simulink model "Inverse_Stewart_Platform_CMM"  (R2024b)
settings: Solver=VariableStepAuto  StartTime=0.0  StopTime=0  RelTol=1e-3
settings Model: Creator=Challa  LastModifiedBy=kodan

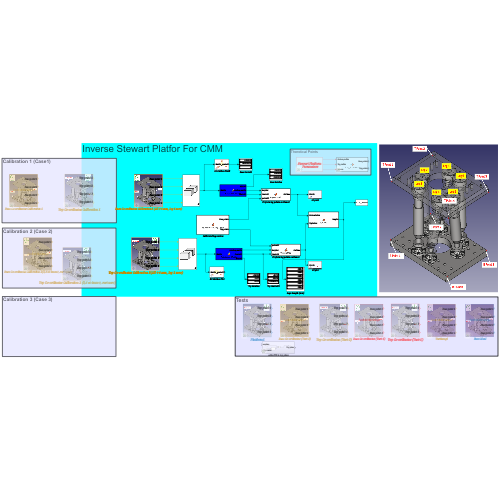
[thumbnail: Simulink's stored preview of the top-level diagram]
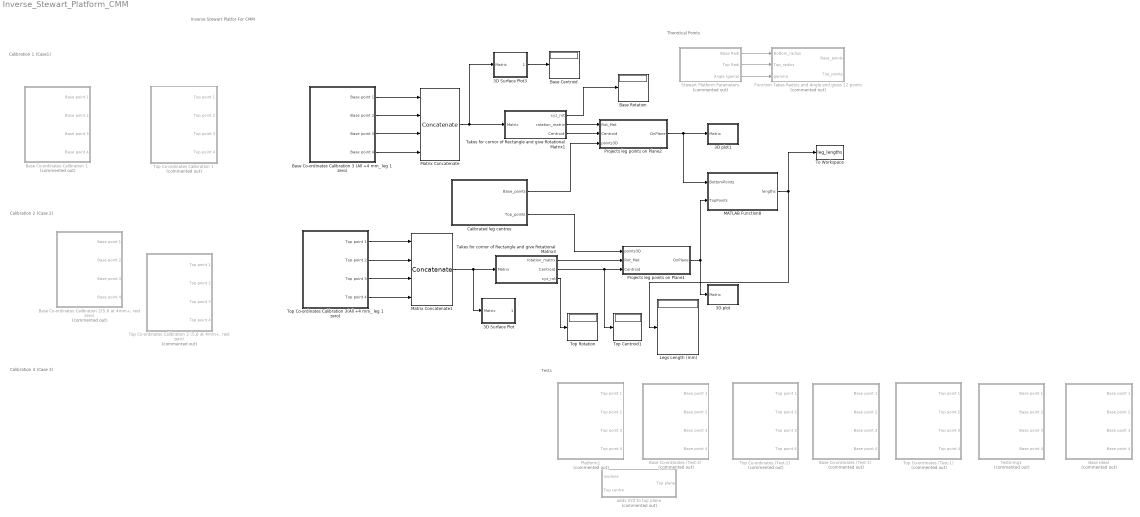
== system Inverse_Stewart_Platform_CMM ==
  note: Therotical Points
  note: Calibration 3 (Case 3)
  note: Inverse Stewart Platfor For CMM
  note: Tests
  note: Calibration 1 (Case1)
  note: Calibration 2 (Case 2)
  3D Surface Plot : Subsystem  mask(3D Surface Plot){color2='r'}
      mask prompts: color2 "color"
      mask help:
      | Input: 3xN matrix
      | output: 3D Surface Plot
      | Color: Changable by giving input
      | Finds Centerpoint and plots.
      mask Help:
      | Input: 3xN matrix
      | output: 3D Surface Plot
      | Color: Changable by giving input
      | Finds Centerpoint and plots.
      mask Display: image('XYZ2.png');
  3D Surface Plot3 : Subsystem  mask(3D Surface Plot){color2='b'}
      mask prompts: color2 "color"
      mask help:
      | Input: 3xN matrix
      | output: 3D Surface Plot
      | Color: Changable by giving input
      | Finds Centerpoint and plots.
      mask Help:
      | Input: 3xN matrix
      | output: 3D Surface Plot
      | Color: Changable by giving input
      | Finds Centerpoint and plots.
      mask Display: image('XYZ2.png');
  3D plot : Subsystem  mask(3D Plot){color1='r'}
      mask prompts: color1 "color"
      mask help:
      | Input: 3xN matrix
      | output: 3D Plot
      | Color: Changable by giving input
      mask Help:
      | Input: 3xN matrix
      | output: 3D Plot
      | Color: Changable by giving input
      mask Display: image('XYZ.png');
  3D plot1 : Subsystem  mask(3D Plot){color1='b'}
      mask prompts: color1 "color"
      mask help:
      | Input: 3xN matrix
      | output: 3D Plot
      | Color: Changable by giving input
      mask Help:
      | Input: 3xN matrix
      | output: 3D Plot
      | Color: Changable by giving input
      mask Display: image('XYZ.png');
  Base Centroid : Display
  Base Co-ordinates (Test-1) : Subsystem  Commented=on  mask(Bottom / Base platform points){B1=[-82.482,112.493,-0.004], B2=[ 82.46,112.505,0.137], B3=[82.505,-112.49,0.004], B4=[-82.482,-112.507,-0.137]}
      mask prompts: B1 "Point 1 [X Y Z] (mm)"; B2 "Point 2 [X Y Z] (mm)"; B3 "Point 3 [X Y Z] (mm)"; B4 "Point 4 [X Y Z] (mm)"
      mask help:
      | Please look at diagram to give Bottom / Base platform points
      | Array [X Y Z] with respect to the Base platform Rectangle centre
      mask Help:
      | Please look at diagram to give Bottom / Base platform points
      | Array [X Y Z] with respect to the Base platform Rectangle centre
      mask Display:
      | disp('Look at the image');
      | image('Screenshot 2024-06-21 170647.png');
  Base Co-ordinates (Test-2) : Subsystem  Commented=on  mask(Bottom / Base platform points){B1=[-82.482,112.494,0.006], B2=[82.459,112.506,0.136], B3=[82.506,-112.491,-0.006], B4=[-82.482,-112.508,-0.136]}
      mask prompts: B1 "Point 1 [X Y Z] (mm)"; B2 "Point 2 [X Y Z] (mm)"; B3 "Point 3 [X Y Z] (mm)"; B4 "Point 4 [X Y Z] (mm)"
      mask help:
      | Please look at diagram to give Bottom / Base platform points
      | Array [X Y Z] with respect to the Base platform Rectangle centre
      mask Help:
      | Please look at diagram to give Bottom / Base platform points
      | Array [X Y Z] with respect to the Base platform Rectangle centre
      mask Display:
      | disp('Look at the image');
      | image('Screenshot 2024-06-21 170647.png');
  Base Co-ordinates Calibration 1 : Subsystem  Commented=on  mask(Bottom / Base platform points){B1=[-82.478,112.495,-0.004], B2=[82.454,112.508,0.112], B3=[82.502,-112.489,0.004], B4=[-82.478,-112.513,-0.112]}
      mask prompts: B1 "Point 1 [X Y Z] (mm)"; B2 "Point 2 [X Y Z] (mm)"; B3 "Point 3 [X Y Z] (mm)"; B4 "Point 4 [X Y Z] (mm)"
      mask help:
      | Please look at diagram to give Bottom / Base platform points
      | Array [X Y Z] with respect to the Base platform Rectangle centre
      mask Help:
      | Please look at diagram to give Bottom / Base platform points
      | Array [X Y Z] with respect to the Base platform Rectangle centre
      mask Display:
      | disp('Look at the image');
      | image('Screenshot 2024-06-21 170647.png');
  "Base Co-ordinates Calibration 2(5,6 at 4mm+, rest zero)" : Subsystem  Commented=on  mask(Bottom / Base platform points){B1=[-82.477,112.496,-0.004], B2=[82.452,112.506,0.125], B3=[82.503,-112.49,0.004], B4=[-82.477,-112.511,-0.125]}
      mask prompts: B1 "Point 1 [X Y Z] (mm)"; B2 "Point 2 [X Y Z] (mm)"; B3 "Point 3 [X Y Z] (mm)"; B4 "Point 4 [X Y Z] (mm)"
      mask help:
      | Please look at diagram to give Bottom / Base platform points
      | Array [X Y Z] with respect to the Base platform Rectangle centre
      mask Help:
      | Please look at diagram to give Bottom / Base platform points
      | Array [X Y Z] with respect to the Base platform Rectangle centre
      mask Display:
      | disp('Look at the image');
      | image('Screenshot 2024-06-21 170647.png');
  Base Co-ordinates Calibration 3 (All +4 mm_ leg 1 zero) : Subsystem  mask(Bottom / Base platform points){B1=[-82.477,112.497,-0.008], B2=[82.453,112.508,0.126], B3=[82.502,-112.492,0.008], B4=[-82.477,-112.513,-0.126]}
      mask prompts: B1 "Point 1 [X Y Z] (mm)"; B2 "Point 2 [X Y Z] (mm)"; B3 "Point 3 [X Y Z] (mm)"; B4 "Point 4 [X Y Z] (mm)"
      mask help:
      | Please look at diagram to give Bottom / Base platform points
      | Array [X Y Z] with respect to the Base platform Rectangle centre
      mask Help:
      | Please look at diagram to give Bottom / Base platform points
      | Array [X Y Z] with respect to the Base platform Rectangle centre
      mask Display:
      | disp('Look at the image');
      | image('Screenshot 2024-06-21 170647.png');
  Base Ideal : Subsystem  Commented=on  mask(Bottom / Base platform points){B1=[-82.5,112.5,0], B2=[82.5,112.5,0], B3=[82.5,-112.5,0], B4=[-82.5,-112.5,0]}
      mask prompts: B1 "Point 1 [X Y Z] (mm)"; B2 "Point 2 [X Y Z] (mm)"; B3 "Point 3 [X Y Z] (mm)"; B4 "Point 4 [X Y Z] (mm)"
      mask help:
      | Please look at diagram to give Bottom / Base platform points
      | Array [X Y Z] with respect to the Base platform Rectangle centre
      mask Help:
      | Please look at diagram to give Bottom / Base platform points
      | Array [X Y Z] with respect to the Base platform Rectangle centre
      mask Display:
      | disp('Look at the image');
      | image('Screenshot 2024-06-21 170647.png');
  Base Rotation : Display
  Calibrated leg centres : MATLAB Function  TreatAsAtomicUnit=on
  Function Takes Radius and Angle and gives 12 points : MATLAB Function  Commented=on  TreatAsAtomicUnit=on
  Legs Length (mm) : Display
  MATLAB Function8 : MATLAB Function  TreatAsAtomicUnit=on
  Matrix Concatenate : Concatenate  NumInputs=4  Mode=Multidimensional array  ConcatenateDimension=2
  Matrix Concatenate1 : Concatenate  NumInputs=4  Mode=Multidimensional array  ConcatenateDimension=2
  Platform1 : Subsystem  Commented=on  mask(Top / Moving Platform Points){T1=|, T2=|, T3=|, T4=|}
      mask T1=|
      | [-122.0492
      | 96.5349
      | 168.8901]
      mask T2=|
      | [27.7169
      | 145.1424
      | 218.2097]
      mask T3=|
      | [102.0492
      | -66.5349
      | 201.1099]
      mask T4=|
      | [-47.7169
      | -115.1424
      | 151.7903]
      mask prompts: T1 "Point 1 [X Y Z] (mm)"; T2 "Point 2 [X Y Z] (mm)"; T3 "Point 3 [X Y Z] (mm)"; T4 "Point 4 [X Y Z] (mm)"
      mask help:
      | Please look at diagram to give Top / Moving Platform points
      | Array [X Y Z] with respect to the Base platform Rectangle centre
      mask Help:
      | Please look at diagram to give Top / Moving Platform points
      | Array [X Y Z] with respect to the Base platform Rectangle centre
      mask Display: image('Screenshot 2024-06-21 172342.png');
  Projects leg points on Plane1 : MATLAB Function  TreatAsAtomicUnit=on
  Projects leg points on Plane2 : MATLAB Function  TreatAsAtomicUnit=on
  Stewart Platform Parameters : Subsystem  Commented=on  mask(Gamma or Angle){B_R=130/2, T_R=125/2, Angle=20}
      mask prompts: B_R "Base Radius (mm)"; T_R "Top Radius(mm)"; Angle "Angle or Gama(deg)"
      mask help: Gamma is the half angle between 2 centres of leg
      mask Help: Gamma is the half angle between 2 centres of leg
      mask Display: disp('Stewart Platform \n Paramaters');
  Takes for cornor of Rectangle and give Rotational Matrix1 : MATLAB Function  TreatAsAtomicUnit=on
  Takes for cornor of Rectangle and give Rotational Matrix3 : MATLAB Function  TreatAsAtomicUnit=on
  Testinmg1 : Subsystem  Commented=on  mask(Bottom / Base platform points){B1=[-82.5,112.5,185], B2=[82.5,112.5,185], B3=[82.5,-112.5,185], B4=[-82.5,-112.5,185]}
      mask prompts: B1 "Point 1 [X Y Z] (mm)"; B2 "Point 2 [X Y Z] (mm)"; B3 "Point 3 [X Y Z] (mm)"; B4 "Point 4 [X Y Z] (mm)"
      mask help:
      | Please look at diagram to give Bottom / Base platform points
      | Array [X Y Z] with respect to the Base platform Rectangle centre
      mask Help:
      | Please look at diagram to give Bottom / Base platform points
      | Array [X Y Z] with respect to the Base platform Rectangle centre
      mask Display:
      | disp('Look at the image');
      | image('Screenshot 2024-06-21 170647.png');
  To Workspace : ToWorkspace  VariableName=leg_lengths  SampleTime=-1
      settings: Save2DSignal=2-D array (concatenate along first dimension)
  Top Centroid1 : Display
  Top Co-ordinates (Test-1) : Subsystem  Commented=on  mask(Top / Moving Platform Points){T1=[-83.589,104.282,181.898], T2=[ 81.27,109.355,180.899], T3=[88.271,-115.398,175.913], T4=[-76.576,-120.558,176.91]}
      mask prompts: T1 "Point 1 [X Y Z] (mm)"; T2 "Point 2 [X Y Z] (mm)"; T3 "Point 3 [X Y Z] (mm)"; T4 "Point 4 [X Y Z] (mm)"
      mask help:
      | Please look at diagram to give Top / Moving Platform points
      | Array [X Y Z] with respect to the Base platform Rectangle centre
      mask Help:
      | Please look at diagram to give Top / Moving Platform points
      | Array [X Y Z] with respect to the Base platform Rectangle centre
      mask Display: image('Screenshot 2024-06-21 172342.png');
  Top Co-ordinates (Test-2) : Subsystem  Commented=on  mask(Top / Moving Platform Points){T1=[-88.819,113.319,179.407], T2=[ 76.042,118.442,180.272], T3=[83.131,-106.372,180.49], T4=[-81.723,-111.564,179.625]}
      mask prompts: T1 "Point 1 [X Y Z] (mm)"; T2 "Point 2 [X Y Z] (mm)"; T3 "Point 3 [X Y Z] (mm)"; T4 "Point 4 [X Y Z] (mm)"
      mask help:
      | Please look at diagram to give Top / Moving Platform points
      | Array [X Y Z] with respect to the Base platform Rectangle centre
      mask Help:
      | Please look at diagram to give Top / Moving Platform points
      | Array [X Y Z] with respect to the Base platform Rectangle centre
      mask Display: image('Screenshot 2024-06-21 172342.png');
  Top Co-ordinates Calibration 1 : Subsystem  Commented=on  mask(Top / Moving Platform Points){T1=[-78.089,115.325,180.165], T2=[86.773,110.209,179.929], T3=[79.912,-114.609,179.521], T4=[-84.943,-109.583,179.756]}
      mask prompts: T1 "Point 1 [X Y Z] (mm)"; T2 "Point 2 [X Y Z] (mm)"; T3 "Point 3 [X Y Z] (mm)"; T4 "Point 4 [X Y Z] (mm)"
      mask help:
      | Please look at diagram to give Top / Moving Platform points
      | Array [X Y Z] with respect to the Base platform Rectangle centre
      mask Help:
      | Please look at diagram to give Top / Moving Platform points
      | Array [X Y Z] with respect to the Base platform Rectangle centre
      mask Display: image('Screenshot 2024-06-21 172342.png');
  "Top Co-ordinates Calibration 2 (5,6 at 4mm+, rest zero)" : Subsystem  Commented=on  mask(Top / Moving Platform Points){T1=[-85.125,127.502,176.101], T2=[79.718,122.365,179.083], T3=[72.703,-102.365,185.192], T4=[-92.131,-97.306,182.212]}
      mask prompts: T1 "Point 1 [X Y Z] (mm)"; T2 "Point 2 [X Y Z] (mm)"; T3 "Point 3 [X Y Z] (mm)"; T4 "Point 4 [X Y Z] (mm)"
      mask help:
      | Please look at diagram to give Top / Moving Platform points
      | Array [X Y Z] with respect to the Base platform Rectangle centre
      mask Help:
      | Please look at diagram to give Top / Moving Platform points
      | Array [X Y Z] with respect to the Base platform Rectangle centre
      mask Display: image('Screenshot 2024-06-21 172342.png');
  Top Co-ordinates Calibration 3(All +4 mm_ leg 1 zero) : Subsystem  mask(Top / Moving Platform Points){T1=[-91.542,118.596,184.014], T2=[73.104,127.707,179.994], T3=[85.709,-96.849,181.665], T4=[-78.923,-106.062,185.686]}
      mask prompts: T1 "Point 1 [X Y Z] (mm)"; T2 "Point 2 [X Y Z] (mm)"; T3 "Point 3 [X Y Z] (mm)"; T4 "Point 4 [X Y Z] (mm)"
      mask help:
      | Please look at diagram to give Top / Moving Platform points
      | Array [X Y Z] with respect to the Base platform Rectangle centre
      mask Help:
      | Please look at diagram to give Top / Moving Platform points
      | Array [X Y Z] with respect to the Base platform Rectangle centre
      mask Display: image('Screenshot 2024-06-21 172342.png');
  Top Rotation : Display
  adds XYZ to top plane : Subsystem  Commented=on
  wires:
  Matrix Concatenate1/1 -> 3D Surface Plot/1(Matrix), Takes for cornor of Rectangle and give Rotational Matrix3/1(Matrix)
  Top Co-ordinates Calibration 3(All +4 mm_ leg 1 zero)/4(Top point 4) -> Matrix Concatenate1/4
  Top Co-ordinates Calibration 3(All +4 mm_ leg 1 zero)/3(Top point 3) -> Matrix Concatenate1/3
  Takes for cornor of Rectangle and give Rotational Matrix1/2(rotation_matrix) -> Projects leg points on Plane2/1(Rot_Mat)
  Top Co-ordinates Calibration 3(All +4 mm_ leg 1 zero)/2(Top point 2) -> Matrix Concatenate1/2
  Takes for cornor of Rectangle and give Rotational Matrix1/3(Centroid) -> Projects leg points on Plane2/2(Centroid)
  Top Co-ordinates Calibration 3(All +4 mm_ leg 1 zero)/1(Top point 1) -> Matrix Concatenate1/1
  Stewart Platform Parameters/3(Angle (gama)) -> Function Takes Radius and Angle and gives 12 points/3(gamma)
  Stewart Platform Parameters/2(Top Radi) -> Function Takes Radius and Angle and gives 12 points/2(Top_radius)
  Stewart Platform Parameters/1(Base Radi) -> Function Takes Radius and Angle and gives 12 points/1(Bottom_radius)
  Calibrated leg centres/1(Base_points) -> Projects leg points on Plane2/3(points3D)
  Calibrated leg centres/2(Top_points) -> Projects leg points on Plane1/1(points3D)
  3D Surface Plot3/1(centroid) -> Base Centroid/1
  Takes for cornor of Rectangle and give Rotational Matrix3/1(rotation_matrix) -> Projects leg points on Plane1/2(Rot_Mat)
  Takes for cornor of Rectangle and give Rotational Matrix3/2(Centroid) -> Projects leg points on Plane1/3(Centroid), Top Centroid1/1
  Base Co-ordinates Calibration 3 (All +4 mm_ leg 1 zero)/4(Base point 4) -> Matrix Concatenate/4
  Takes for cornor of Rectangle and give Rotational Matrix3/3(xyz_rot) -> Top Rotation/1
  Projects leg points on Plane2/1(OnPlane) -> MATLAB Function8/1(BottomPoints), 3D plot1/1(Matrix)
  Projects leg points on Plane1/1(OnPlane) -> MATLAB Function8/2(TopPoints), 3D plot/1(Matrix)
  MATLAB Function8/1(lengths) -> Legs Length (mm)/1, To Workspace/1
  Base Co-ordinates Calibration 3 (All +4 mm_ leg 1 zero)/1(Base point 1) -> Matrix Concatenate/1
  Base Co-ordinates Calibration 3 (All +4 mm_ leg 1 zero)/2(Base point 2) -> Matrix Concatenate/2
  Base Co-ordinates Calibration 3 (All +4 mm_ leg 1 zero)/3(Base point 3) -> Matrix Concatenate/3
  Matrix Concatenate/1 -> 3D Surface Plot3/1(Matrix), Takes for cornor of Rectangle and give Rotational Matrix1/1(Matrix)
  Takes for cornor of Rectangle and give Rotational Matrix1/1(xyz_rot) -> Base Rotation/1

== system Inverse_Stewart_Platform_CMM/3D Surface Plot ==
  Matrix : Inport
  MATLAB Function6 : MATLAB Function  TreatAsAtomicUnit=on
  Plot3D1 : MATLAB Function  TreatAsAtomicUnit=on
  Plot3D6 : MATLAB Function  TreatAsAtomicUnit=on
  String Constant : StringConstant  String=color2
  centroid : Outport
  wires:
  Matrix/1 -> Plot3D1/1(Matrix), MATLAB Function6/1(Matrix)
  MATLAB Function6/1(centroid) -> centroid/1, Plot3D6/1(Matrix)
  String Constant/1 -> Plot3D6/2(color2), Plot3D1/2(color2)

== system Inverse_Stewart_Platform_CMM/3D Surface Plot3 ==
  Matrix : Inport
  MATLAB Function6 : MATLAB Function  TreatAsAtomicUnit=on
  Plot3D1 : MATLAB Function  TreatAsAtomicUnit=on
  Plot3D6 : MATLAB Function  TreatAsAtomicUnit=on
  String Constant : StringConstant  String=color2
  centroid : Outport
  wires:
  String Constant/1 -> Plot3D1/2(color2), Plot3D6/2(color2)
  MATLAB Function6/1(centroid) -> Plot3D6/1(Matrix), centroid/1
  Matrix/1 -> MATLAB Function6/1(Matrix), Plot3D1/1(Matrix)

== system Inverse_Stewart_Platform_CMM/3D plot ==
  Matrix : Inport
  Plot3D1 : MATLAB Function  TreatAsAtomicUnit=on
  String Constant : StringConstant  String=color1
  wires:
  String Constant/1 -> Plot3D1/2(color1)
  Matrix/1 -> Plot3D1/1(Matrix)

== system Inverse_Stewart_Platform_CMM/3D plot1 ==
  Matrix : Inport
  Plot3D1 : MATLAB Function  TreatAsAtomicUnit=on
  String Constant : StringConstant  String=color1
  wires:
  Matrix/1 -> Plot3D1/1(Matrix)
  String Constant/1 -> Plot3D1/2(color1)

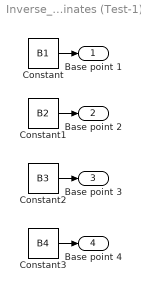
== system Inverse_Stewart_Platform_CMM/Base Co-ordinates (Test-1) ==
  Constant : Constant  Value=B1
  Constant1 : Constant  Value=B2
  Constant2 : Constant  Value=B3
  Constant3 : Constant  Value=B4
  Base point 1 : Outport
  Base point 2 : Outport  Port=2
  Base point 3 : Outport  Port=3
  Base point 4 : Outport  Port=4
  wires:
  Constant1/1 -> Base point 2/1
  Constant3/1 -> Base point 4/1
  Constant2/1 -> Base point 3/1
  Constant/1 -> Base point 1/1

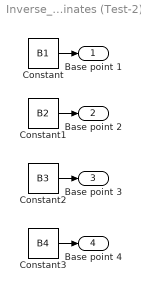
== system Inverse_Stewart_Platform_CMM/Base Co-ordinates (Test-2) ==
  Constant : Constant  Value=B1
  Constant1 : Constant  Value=B2
  Constant2 : Constant  Value=B3
  Constant3 : Constant  Value=B4
  Base point 1 : Outport
  Base point 2 : Outport  Port=2
  Base point 3 : Outport  Port=3
  Base point 4 : Outport  Port=4
  wires:
  Constant1/1 -> Base point 2/1
  Constant3/1 -> Base point 4/1
  Constant2/1 -> Base point 3/1
  Constant/1 -> Base point 1/1

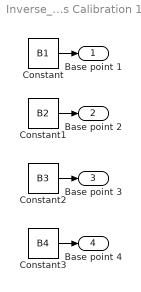
== system Inverse_Stewart_Platform_CMM/Base Co-ordinates Calibration 1 ==
  Constant : Constant  Value=B1
  Constant1 : Constant  Value=B2
  Constant2 : Constant  Value=B3
  Constant3 : Constant  Value=B4
  Base point 1 : Outport
  Base point 2 : Outport  Port=2
  Base point 3 : Outport  Port=3
  Base point 4 : Outport  Port=4
  wires:
  Constant/1 -> Base point 1/1
  Constant2/1 -> Base point 3/1
  Constant3/1 -> Base point 4/1
  Constant1/1 -> Base point 2/1

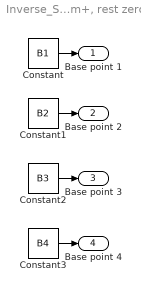
== system Inverse_Stewart_Platform_CMM/Base Co-ordinates Calibration 2(5,6 at 4mm+, rest zero) ==
  Constant : Constant  Value=B1
  Constant1 : Constant  Value=B2
  Constant2 : Constant  Value=B3
  Constant3 : Constant  Value=B4
  Base point 1 : Outport
  Base point 2 : Outport  Port=2
  Base point 3 : Outport  Port=3
  Base point 4 : Outport  Port=4
  wires:
  Constant1/1 -> Base point 2/1
  Constant3/1 -> Base point 4/1
  Constant2/1 -> Base point 3/1
  Constant/1 -> Base point 1/1

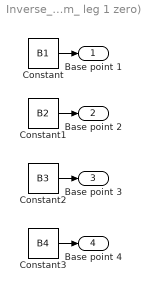
== system Inverse_Stewart_Platform_CMM/Base Co-ordinates Calibration 3 (All +4 mm_ leg 1 zero) ==
  Constant : Constant  Value=B1
  Constant1 : Constant  Value=B2
  Constant2 : Constant  Value=B3
  Constant3 : Constant  Value=B4
  Base point 1 : Outport
  Base point 2 : Outport  Port=2
  Base point 3 : Outport  Port=3
  Base point 4 : Outport  Port=4
  wires:
  Constant1/1 -> Base point 2/1
  Constant3/1 -> Base point 4/1
  Constant2/1 -> Base point 3/1
  Constant/1 -> Base point 1/1

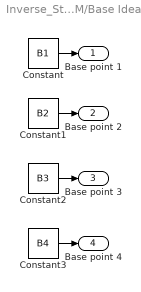
== system Inverse_Stewart_Platform_CMM/Base Ideal ==
  Constant : Constant  Value=B1
  Constant1 : Constant  Value=B2
  Constant2 : Constant  Value=B3
  Constant3 : Constant  Value=B4
  Base point 1 : Outport
  Base point 2 : Outport  Port=2
  Base point 3 : Outport  Port=3
  Base point 4 : Outport  Port=4
  wires:
  Constant/1 -> Base point 1/1
  Constant2/1 -> Base point 3/1
  Constant3/1 -> Base point 4/1
  Constant1/1 -> Base point 2/1

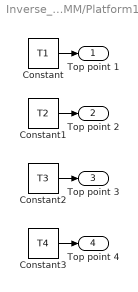
== system Inverse_Stewart_Platform_CMM/Platform1 ==
  Constant : Constant  Value=T1
  Constant1 : Constant  Value=T2
  Constant2 : Constant  Value=T3
  Constant3 : Constant  Value=T4
  Top point 1 : Outport
  Top point 2 : Outport  Port=2
  Top point 3 : Outport  Port=3
  Top point 4 : Outport  Port=4
  wires:
  Constant/1 -> Top point 1/1
  Constant2/1 -> Top point 3/1
  Constant3/1 -> Top point 4/1
  Constant1/1 -> Top point 2/1

== system Inverse_Stewart_Platform_CMM/Stewart Platform Parameters ==
  Angle : Constant  Value=Angle
  Base Radius : Constant  Value=B_R
  Top Radius : Constant  Value=T_R
  Base Radi : Outport
  Top Radi : Outport  Port=2
  Angle (gama) : Outport  Port=3
  wires:
  Angle/1 -> Angle (gama)/1
  Base Radius/1 -> Base Radi/1
  Top Radius/1 -> Top Radi/1

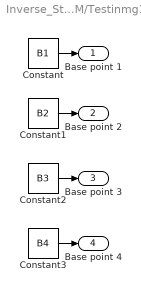
== system Inverse_Stewart_Platform_CMM/Testinmg1 ==
  Constant : Constant  Value=B1
  Constant1 : Constant  Value=B2
  Constant2 : Constant  Value=B3
  Constant3 : Constant  Value=B4
  Base point 1 : Outport
  Base point 2 : Outport  Port=2
  Base point 3 : Outport  Port=3
  Base point 4 : Outport  Port=4
  wires:
  Constant1/1 -> Base point 2/1
  Constant3/1 -> Base point 4/1
  Constant2/1 -> Base point 3/1
  Constant/1 -> Base point 1/1

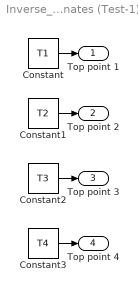
== system Inverse_Stewart_Platform_CMM/Top Co-ordinates (Test-1) ==
  Constant : Constant  Value=T1
  Constant1 : Constant  Value=T2
  Constant2 : Constant  Value=T3
  Constant3 : Constant  Value=T4
  Top point 1 : Outport
  Top point 2 : Outport  Port=2
  Top point 3 : Outport  Port=3
  Top point 4 : Outport  Port=4
  wires:
  Constant1/1 -> Top point 2/1
  Constant3/1 -> Top point 4/1
  Constant2/1 -> Top point 3/1
  Constant/1 -> Top point 1/1

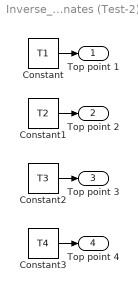
== system Inverse_Stewart_Platform_CMM/Top Co-ordinates (Test-2) ==
  Constant : Constant  Value=T1
  Constant1 : Constant  Value=T2
  Constant2 : Constant  Value=T3
  Constant3 : Constant  Value=T4
  Top point 1 : Outport
  Top point 2 : Outport  Port=2
  Top point 3 : Outport  Port=3
  Top point 4 : Outport  Port=4
  wires:
  Constant/1 -> Top point 1/1
  Constant2/1 -> Top point 3/1
  Constant3/1 -> Top point 4/1
  Constant1/1 -> Top point 2/1

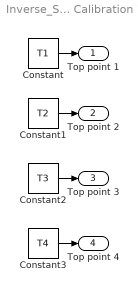
== system Inverse_Stewart_Platform_CMM/Top Co-ordinates Calibration 1 ==
  Constant : Constant  Value=T1
  Constant1 : Constant  Value=T2
  Constant2 : Constant  Value=T3
  Constant3 : Constant  Value=T4
  Top point 1 : Outport
  Top point 2 : Outport  Port=2
  Top point 3 : Outport  Port=3
  Top point 4 : Outport  Port=4
  wires:
  Constant1/1 -> Top point 2/1
  Constant3/1 -> Top point 4/1
  Constant2/1 -> Top point 3/1
  Constant/1 -> Top point 1/1

== system Inverse_Stewart_Platform_CMM/Top Co-ordinates Calibration 2 (5,6 at 4mm+, rest zero) ==
  Constant : Constant  Value=T1
  Constant1 : Constant  Value=T2
  Constant2 : Constant  Value=T3
  Constant3 : Constant  Value=T4
  Top point 1 : Outport
  Top point 2 : Outport  Port=2
  Top point 3 : Outport  Port=3
  Top point 4 : Outport  Port=4
  wires:
  Constant/1 -> Top point 1/1
  Constant2/1 -> Top point 3/1
  Constant3/1 -> Top point 4/1
  Constant1/1 -> Top point 2/1

== system Inverse_Stewart_Platform_CMM/Top Co-ordinates Calibration 3(All +4 mm_ leg 1 zero) ==
  Constant : Constant  Value=T1
  Constant1 : Constant  Value=T2
  Constant2 : Constant  Value=T3
  Constant3 : Constant  Value=T4
  Top point 1 : Outport
  Top point 2 : Outport  Port=2
  Top point 3 : Outport  Port=3
  Top point 4 : Outport  Port=4
  wires:
  Constant/1 -> Top point 1/1
  Constant2/1 -> Top point 3/1
  Constant3/1 -> Top point 4/1
  Constant1/1 -> Top point 2/1

== system Inverse_Stewart_Platform_CMM/adds XYZ to top plane ==
  onplane : Inport
  " Top centre" : Inport  Port=2
  Add : Sum
  MATLAB Function : MATLAB Function  TreatAsAtomicUnit=on
  Top plane : Outport
  wires:
  onplane/1 -> Add/1
  " Top centre"/1 -> MATLAB Function/1(u)
  Add/1 -> Top plane/1
  MATLAB Function/1(y) -> Add/2

== matlab function Inverse_Stewart_Platform_CMM/3D Surface Plot/Plot3D6 ==
  data: Matrix input; color2 input
function Plot3D(Matrix,color2)

figure(1)
x = Matrix(1, :);
y = Matrix(2, :);
z = Matrix(3, :);

% Create the 3D plot
plot3(x, y, z, 'o-', 'Color',color2,'LineWidth', 2);

xlabel('X Axis');
ylabel('Y Axis');
zlabel('Z Axis');


grid on


hold on;

% Connect the initial and final points
plot3([x(1) x(end)], [y(1) y(end)], [z(1) z(end)], 'o-', 'Color',color2,'LineWidth', 2);

%hold on

end

== matlab function Inverse_Stewart_Platform_CMM/Takes for cornor of Rectangle and give Rotational Matrix3 ==
  data: Matrix input; rotation_matrix output; Centroid output; xyz_rot output
function [rotation_matrix,Centroid, xyz_rot] = Rotational_Matrix(Matrix)
    % A, B, C, D are the 3D coordinates of the rectangle's corners

    Centroid = mean(Matrix, 2);

    A = Matrix(:,1);
    B = Matrix(:,2);
    C = Matrix(:,3);
    D = Matrix(:,4);

    % Calculate the normal vector of the plane using cross product
    AB = B - A;
    AD = A - D;
    normal = cross(AB, AD);
    normal = normal / norm(normal); % Normalize the normal vector

    % Create orthogonal basis vectors on the plane
    e1 = AB / norm(AB); % First direction vector on the plane
    e2 = cross(normal, e1); % Second direction vector on the plane

    % Construct the rotation matrix from the plane's basis vectors
    rotation_matrix = [e1 e2 normal];

    % Calculate Euler angles (rotations in XYZ)
    xyz_rot = rad2deg(rotm2eul(rotation_matrix,"XYZ"));


    % Assuming the rectangle is initially aligned with the XY plane,
    % we can calculate the rotations needed to align it with the given orientation.
    % % % % % thetaX = atan2(normal(2), normal(3));
    % % % % % thetaY = atan2(-normal(1), sqrt(normal(2)^2 + normal(3)^2));
    % % % % % thetaZ = atan2(AB(2), AB(1));
    % % % % % 
    % % % % % % Convert angles to degrees
    % % % % % thetaX_deg = rad2deg(thetaX);
    % % % % % thetaY_deg = rad2deg(thetaY);
    % % % % % thetaZ_deg = rad2deg(thetaZ);
    % % % % % xyz_rot = [thetaX_deg,thetaY_deg, thetaZ_deg];
end

== matlab function Inverse_Stewart_Platform_CMM/3D Surface Plot3/MATLAB Function6 ==
  data: Matrix input; centroid output
function centroid  = FindCentroid(Matrix)
    % This function calculates the centroid of a 3xN matrix
    % points: a 3xN matrix where each column represents a point in 3D space
    % centroid: a 3x1 vector representing the center point of the given points

    % Validate input
    if size(Matrix, 1) ~= 3
        error('Input matrix must have 3 rows');
    end

    % Calculate the centroid
    centroid = mean(Matrix, 2);
end

== matlab function Inverse_Stewart_Platform_CMM/3D Surface Plot3/Plot3D1 ==
  data: Matrix input; color2 input
function Plot3D(Matrix, color2)

figure(1)
x = Matrix(1, :);
y = Matrix(2, :);
z = Matrix(3, :);

% Create the 3D plot
plot3(x, y, z, 'o-', 'Color',color2,'LineWidth', 2);
hold on
fill3(x, y, z, color2, 'FaceAlpha', 0.2)
xlabel('X Axis');
ylabel('Y Axis');
zlabel('Z Axis');

axis equal
grid on


hold on;

% Connect the initial and final points
plot3([x(1) x(end)], [y(1) y(end)], [z(1) z(end)], 'o-', 'Color',color2,'LineWidth', 2);

hold on

end

== matlab function Inverse_Stewart_Platform_CMM/3D Surface Plot3/Plot3D6 ==
  data: Matrix input; color2 input
function Plot3D(Matrix,color2)

figure(1)
x = Matrix(1, :);
y = Matrix(2, :);
z = Matrix(3, :);

% Create the 3D plot
plot3(x, y, z, 'o-', 'Color',color2,'LineWidth', 2);
xlabel('X Axis');
ylabel('Y Axis');
zlabel('Z Axis');


grid on


hold on;

% Connect the initial and final points
plot3([x(1) x(end)], [y(1) y(end)], [z(1) z(end)], 'o-', 'Color',color2,'LineWidth', 2);

hold on

end

== matlab function Inverse_Stewart_Platform_CMM/adds XYZ to top plane/MATLAB Function ==
  data: u input; y output
function y = reshape_matrix(u)
    y = repmat(u, 1, 6); % Replicate the 3x1 matrix into a 3x6 matrix
end

== matlab function Inverse_Stewart_Platform_CMM/Function Takes Radius and Angle and gives 12 points ==
  data: Bottom_radius input; Base_points output; Top_radius input; gamma input; Top_points output
function [Base_points, Top_points]= Leg_locations(Bottom_radius, Top_radius, gamma)
    % Define the fixed and moving platform geometry (attachment points)
    % Fixed platform attachment points (in the base frame)
    r1 = Bottom_radius;
    r2 = Top_radius;
    A0=[r1*cosd(60-gamma) r1*sind(60-gamma) 0]'; 
    B0=[r1*cosd(60+gamma) r1*sind(60+gamma) 0]'; 
    C0=[-r1*cosd(gamma) r1*sind(gamma) 0]'; 
    D0=[-r1*cosd(gamma) -r1*sind(gamma) 0]'; 
    E0=[r1*cosd(60+gamma) -r1*sind(60+gamma) 0]'; 
    F0=[r1*cosd(60-gamma) -r1*sind(60-gamma) 0]'; 
    
    B = [A0 B0 C0 D0 E0 F0];
    
    % Moving platform attachment points (in the moving frame)
    
    A1=[r2*cosd(gamma) r2*sind(gamma) 0]';
    B1=[-r2*sind(30-gamma) r2*cosd(30-gamma) 0]';
    C1=[-r2*sind(30+gamma) r2*cosd(30+gamma) 0]';
    D1=[-r2*sind(30+gamma) -r2*cosd(30+gamma) 0]';
    E1=[-r2*sind(30-gamma) -r2*cosd(30-gamma) 0]';
    F1=[r2*cosd(gamma) -r2*sind(gamma) 0]';
    
    P = [A1 B1 C1 D1 E1 F1];
    
Base_points  = B;
Top_points = P;

== matlab function Inverse_Stewart_Platform_CMM/3D plot/Plot3D1 ==
  data: Matrix input; color1 input
function Plot3D(Matrix,color1)

figure(1)
x = Matrix(1, :);
y = Matrix(2, :);
z = Matrix(3, :);

% Create the 3D plot
plot3(x, y, z, 'o-', 'color',color1,'LineWidth', 2);
xlabel('X Axis');
ylabel('Y Axis');
zlabel('Z Axis');

axis equal
grid on


hold on;

% Connect the initial and final points
plot3([x(1) x(end)], [y(1) y(end)], [z(1) z(end)], 'o-', 'Color',color1,'LineWidth', 2);

hold on

end

== matlab function Inverse_Stewart_Platform_CMM/3D plot1/Plot3D1 ==
  data: Matrix input; color1 input
function Plot3D(Matrix,color1)

figure(1)
x = Matrix(1, :);
y = Matrix(2, :);
z = Matrix(3, :);

% Create the 3D plot
plot3(x, y, z, 'o-', 'color',color1,'LineWidth', 2);
xlabel('X Axis');
ylabel('Y Axis');
zlabel('Z Axis');

axis equal
grid on


hold on;

% Connect the initial and final points
plot3([x(1) x(end)], [y(1) y(end)], [z(1) z(end)], 'o-', 'Color',color1,'LineWidth', 2);

hold on

end

== matlab function Inverse_Stewart_Platform_CMM/Takes for cornor of Rectangle and give Rotational Matrix1 ==
  data: xyz_rot output; Matrix input; rotation_matrix output; Centroid output
function [xyz_rot, rotation_matrix,Centroid] = Rotational_Matrix(Matrix)
    % A, B, C, D are the 3D coordinates of the rectangle's corners

    Centroid = mean(Matrix, 2);

    A = Matrix(:,1);
    B = Matrix(:,2);
    C = Matrix(:,3);
    D = Matrix(:,4);

    % Calculate the normal vector of the plane using cross product
    AB = B - A;
    AD = A - D;
    normal = cross(AB, AD);
    normal = normal / norm(normal); % Normalize the normal vector

    % Create orthogonal basis vectors on the plane
    e1 = AB / norm(AB); % First direction vector on the plane
    e2 = cross(normal, e1); % Second direction vector on the plane

    % Construct the rotation matrix from the plane's basis vectors
    rotation_matrix = [e1 e2 normal];

    % Calculate Euler angles (rotations in XYZ)
    xyz_rot = rad2deg(rotm2eul(rotation_matrix,"XYZ"));


    % Assuming the rectangle is initially aligned with the XY plane,
    % we can calculate the rotations needed to align it with the given orientation.
    % % % % % thetaX = atan2(normal(2), normal(3));
    % % % % % thetaY = atan2(-normal(1), sqrt(normal(2)^2 + normal(3)^2));
    % % % % % thetaZ = atan2(AB(2), AB(1));
    % % % % % 
    % % % % % % Convert angles to degrees
    % % % % % thetaX_deg = rad2deg(thetaX);
    % % % % % thetaY_deg = rad2deg(thetaY);
    % % % % % thetaZ_deg = rad2deg(thetaZ);
    % % % % % xyz_rot = [thetaX_deg,thetaY_deg, thetaZ_deg];
end

== matlab function Inverse_Stewart_Platform_CMM/Projects leg points on Plane2 ==
  data: Rot_Mat input; OnPlane output; Centroid input; points3D input
function OnPlane  = ProjectOn3D( Rot_Mat,  Centroid, points3D)
    % Project points onto the XY plane in 3D
    
    % Perform the projection
    OnPlane = Rot_Mat * points3D +  Centroid;
end

== matlab function Inverse_Stewart_Platform_CMM/Calibrated leg centres ==
  data: Base_points output; Top_points output
function [ Base_points, Top_points]= Leg_locations_Top_Base
    % Define the fixed and moving platform geometry (attachment points)
    % Fixed platform attachment points (in the base frame)
    B1=[49.834,41.765,-10.52+11]'; 
    B2=[11.327,63.988,-10.504+11]'; 
    B3=[-61.058, 22.228,-10.654+11]'; 
    B4=[-61.06,-22.233,-10.803+11]'; 
    B5=[11.3,-64.009,-10.898+11]'; 
    B6=[49.825,-41.784,-10.779+11]'; 
    
    B = [B1 B2 B3 B4 B5 B6];
    
    % Moving platform attachment points (in the moving frame)
    
    %%% Actual Top Points
    P1=[58.708,21.383,-11.171+11]';
    P2=[-10.875,61.556,-10.94+11]';
    P3=[-47.912,40.187,-10.888+11]';
    P4=[-47.907,-40.162,-11.017+11]';
    P5=[-10.873,-61.536,-11.135+11]';
    P6=[58.704,-21.364,-11.243+11]';
    
    P = [P1 P2 P3 P4 P5 P6];
    
Base_points  = B;
Top_points = P;

== matlab function Inverse_Stewart_Platform_CMM/3D Surface Plot/MATLAB Function6 ==
  data: Matrix input; centroid output
function centroid  = FindCentroid(Matrix)
    % This function calculates the centroid of a 3xN matrix
    % points: a 3xN matrix where each column represents a point in 3D space
    % centroid: a 3x1 vector representing the center point of the given points

    % Validate input
    if size(Matrix, 1) ~= 3
        error('Input matrix must have 3 rows');
    end

    % Calculate the centroid
    centroid = mean(Matrix, 2);
end

== matlab function Inverse_Stewart_Platform_CMM/3D Surface Plot/Plot3D1 ==
  data: Matrix input; color2 input
function Plot3D(Matrix, color2)

figure(1)
x = Matrix(1, :);
y = Matrix(2, :);
z = Matrix(3, :);

% Create the 3D plot
plot3(x, y, z, 'o-', 'Color',color2,'LineWidth', 2);
hold on
fill3(x, y, z, color2, 'FaceAlpha', 0.2)
xlabel('X Axis');
ylabel('Y Axis');
zlabel('Z Axis');

axis equal
grid on


hold on;

% Connect the initial and final points
plot3([x(1) x(end)], [y(1) y(end)], [z(1) z(end)], 'o-', 'Color',color2,'LineWidth', 2);

hold on

end

== matlab function Inverse_Stewart_Platform_CMM/Projects leg points on Plane1 ==
  data: points3D input; Rot_Mat input; OnPlane output; Centroid input
function OnPlane  = ProjectOn3D( points3D, Rot_Mat,  Centroid)
    % Project points onto the XY plane in 3D
    
    % Perform the projection
    OnPlane = Rot_Mat * points3D +  Centroid;
end

== matlab function Inverse_Stewart_Platform_CMM/MATLAB Function8 ==
  data: BottomPoints input; TopPoints input; lengths output
function lengths = Legs_Plot( BottomPoints, TopPoints)

    % Plotting legs
    figure(1)
    count = 0;
    while count < 6
        count = count + 1;  % Increment the counter
        i = count;
        % Create the 3D plot
        plot3([TopPoints(1,i) BottomPoints(1,i)], [TopPoints(2,i) BottomPoints(2,i)], [TopPoints(3,i) BottomPoints(3,i)], 'Color','g','LineWidth', 2);
        hold on
    end
lengths = [0 0 0 0 0 0];
count = 0;
    while count < 6
        count = count + 1;  % Increment the counter
        i = count;
        % Create the 3D plot
        d = sqrt((TopPoints(1,i) - BottomPoints(1,i))^2 + (TopPoints(2,i)-BottomPoints(2,i))^2 + (TopPoints(3,i) - BottomPoints(3,i))^2);
        lengths(i) = d;
    end
end
